simulink model "gm_I2S"  (R2023b)
settings: Solver=VariableStepAuto  StartTime=0.0  StopTime=10000  RelTol=1e-3
undefined symbols (not defined in the file or in its folder): cnt1_LRCLK, cnt2_SCLK, SH_R
libraries: hdlsllib x10
(part 1 of 5)
settings Model: Creator=31651  LastModifiedBy=31651
settings OptimizationCC: BlockReduction=off  ConditionallyExecuteInputs=off  DefaultParameterBehavior=Inlined
settings DebuggingCC: AlgebraicLoopMsg=error  InheritedTsInSrcMsg=none  ParameterPrecisionLossMsg=none
settings HardwareCC: ProdBitPerPointer=32  ProdBitPerSizeT=32  ProdBitPerPtrDiffT=32  ProdLargestAtomicFloat=None  ProdIntDivRoundTo=Undefined  ProdEndianess=Unspecified  ProdWordSize=32  ProdHWDeviceType=ASIC/FPGA->ASIC/FPGA  TargetBitPerPointer=64  TargetBitPerSizeT=64  TargetBitPerPtrDiffT=64  TargetLongLongMode=on  TargetIntDivRoundTo=Zero  TargetEndianess=LittleEndian  TargetWordSize=64  TargetHWDeviceType=Custom Processor->MATLAB Host Computer  ProdEqTarget=off

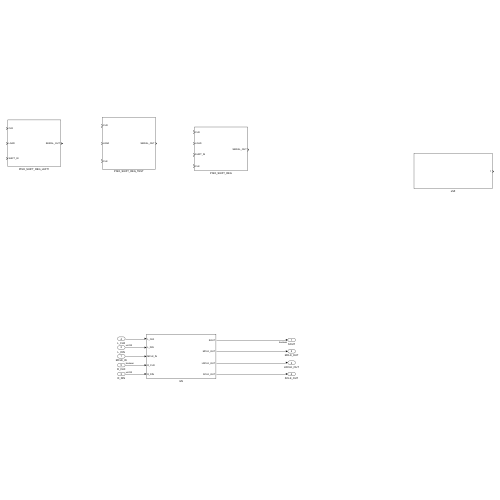
[thumbnail: Simulink's stored preview of the top-level diagram]
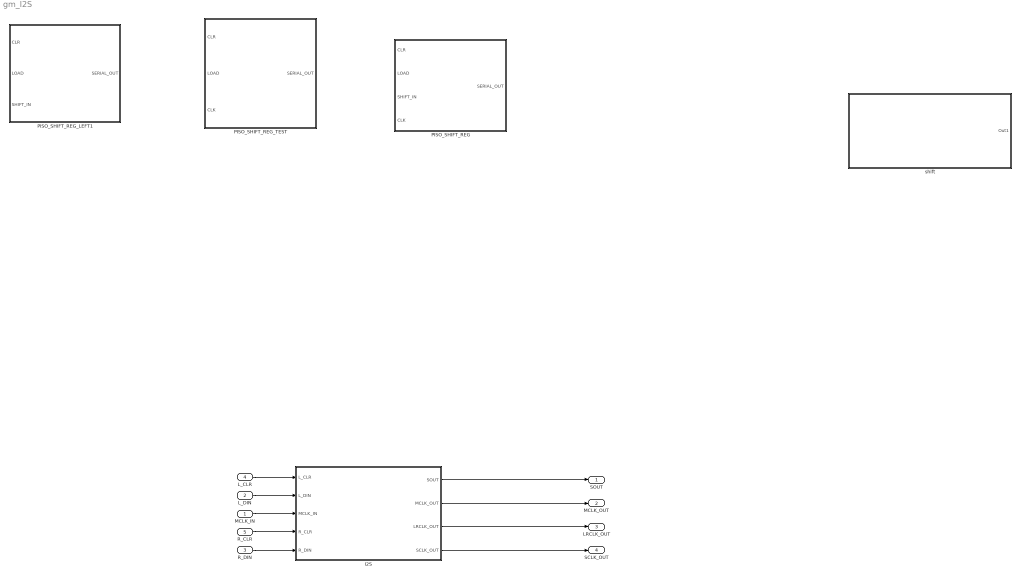
== system gm_I2S ==
  MCLK_IN : Inport
  L_DIN : Inport  Port=2  OutDataTypeStr=uint32
  R_DIN : Inport  Port=3  OutDataTypeStr=uint32
  L_CLR : Inport  Port=4
  R_CLR : Inport  Port=5  OutDataTypeStr=boolean
  I2S : Subsystem
  PISO_SHIFT_REG : Subsystem
  PISO_SHIFT_REG_LEFT1 : Subsystem
  PISO_SHIFT_REG_TEST : Subsystem
  shift : Subsystem
  SOUT : Outport  OutDataTypeStr=boolean  VectorParamsAs1DForOutWhenUnconnected=off
  MCLK_OUT : Outport  Port=2  VectorParamsAs1DForOutWhenUnconnected=off
  LRCLK_OUT : Outport  Port=3  VectorParamsAs1DForOutWhenUnconnected=off
  SCLK_OUT : Outport  Port=4  VectorParamsAs1DForOutWhenUnconnected=off
  wires:
  R_CLR/1 -> I2S/4(R_CLR)
  L_CLR/1 -> I2S/1(L_CLR)
  I2S/4(SCLK_OUT) -> SCLK_OUT/1
  I2S/3(LRCLK_OUT) -> LRCLK_OUT/1
  I2S/2(MCLK_OUT) -> MCLK_OUT/1
  I2S/1(SOUT) -> SOUT/1
  R_DIN/1 -> I2S/5(R_DIN)
  MCLK_IN/1 -> I2S/3(MCLK_IN)
  L_DIN/1 -> I2S/2(L_DIN)

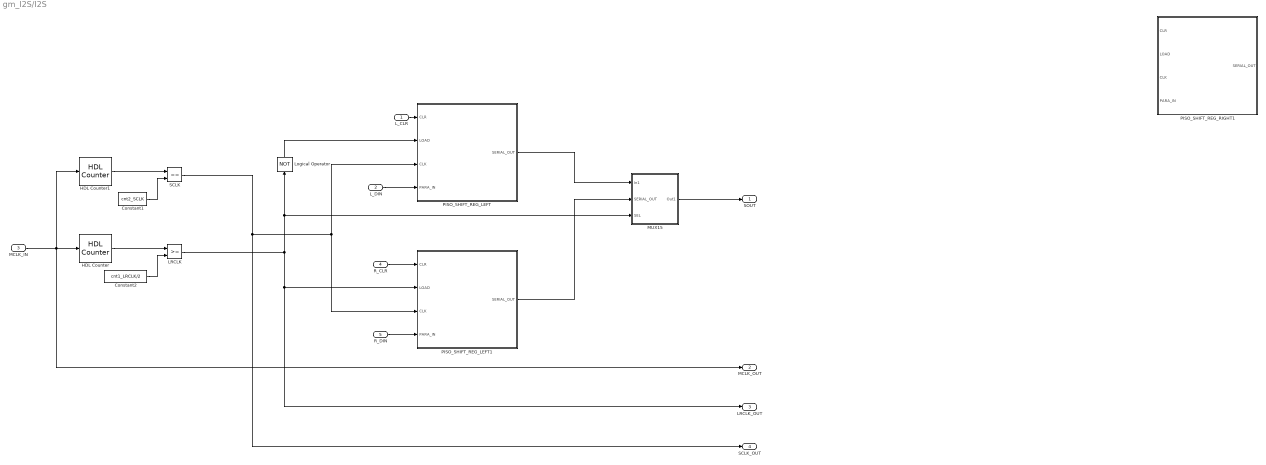
== system gm_I2S/I2S ==
  L_CLR : Inport
  L_DIN : Inport  Port=2
  MCLK_IN : Inport  Port=3
  R_CLR : Inport  Port=4
  R_DIN : Inport  Port=5
  Constant1 : Constant  Value=cnt2_SCLK  OutDataTypeStr=uint16
  Constant2 : Constant  Value=cnt1_LRCLK/2  OutDataTypeStr=uint16
  HDL Counter : hdlsllib/Sources/HDL Counter  CountType=Count limited  CountInit=0  CountStep=1  CountMax=cnt1_LRCLK  CountFromType=Initial value  CountFrom=0  CountResetPort=off  CountLoadPort=off  CountEnbPort=on  CountDirPort=off  CountHitOutputPort=off  CountDataType=Unsigned  CountWordLen=16  CountFracLen=0  CountSampTime=1
  HDL Counter1 : hdlsllib/Sources/HDL Counter  CountType=Count limited  CountInit=0  CountStep=1  CountMax=cnt2_SCLK  CountFromType=Initial value  CountFrom=0  CountResetPort=off  CountLoadPort=off  CountEnbPort=on  CountDirPort=off  CountHitOutputPort=off  CountDataType=Unsigned  CountWordLen=16  CountFracLen=0  CountSampTime=1
  LRCLK : RelationalOperator  OutDataTypeStr=boolean  InputSameDT=off
  Logical Operator : Logic  Operator=NOT  AllPortsSameDT=off  OutDataTypeStr=boolean
  MUX15 : Subsystem
  PISO_SHIFT_REG_LEFT : Subsystem
  PISO_SHIFT_REG_LEFT1 : Subsystem
  PISO_SHIFT_REG_RIGHT1 : Subsystem
  SCLK : RelationalOperator  Operator===  OutDataTypeStr=boolean  InputSameDT=off
  SOUT : Outport  VectorParamsAs1DForOutWhenUnconnected=off
  MCLK_OUT : Outport  Port=2  VectorParamsAs1DForOutWhenUnconnected=off
  LRCLK_OUT : Outport  Port=3  VectorParamsAs1DForOutWhenUnconnected=off
  SCLK_OUT : Outport  Port=4  VectorParamsAs1DForOutWhenUnconnected=off
  wires:
  L_DIN/1 -> PISO_SHIFT_REG_LEFT/4(PARA_IN)
  R_DIN/1 -> PISO_SHIFT_REG_LEFT1/4(PARA_IN)
  L_CLR/1 -> PISO_SHIFT_REG_LEFT/1(CLR)
  Constant2/1 -> LRCLK/2
  HDL Counter1/1 -> SCLK/1
  R_CLR/1 -> PISO_SHIFT_REG_LEFT1/1(CLR)
  MUX15/1(Out1) -> SOUT/1
  Constant1/1 -> SCLK/2
  PISO_SHIFT_REG_LEFT1/1(SERIAL_OUT) -> MUX15/2(SERIAL_OUT)
  MCLK_IN/1 -> HDL Counter/1, HDL Counter1/1, MCLK_OUT/1
  HDL Counter/1 -> LRCLK/1
  PISO_SHIFT_REG_LEFT/1(SERIAL_OUT) -> MUX15/1(In1)
  LRCLK/1 -> MUX15/3(SEL), Logical Operator/1, LRCLK_OUT/1, PISO_SHIFT_REG_LEFT1/2(LOAD)
  Logical Operator/1 -> PISO_SHIFT_REG_LEFT/2(LOAD)
  SCLK/1 -> PISO_SHIFT_REG_LEFT/3(CLK), PISO_SHIFT_REG_LEFT1/3(CLK), SCLK_OUT/1

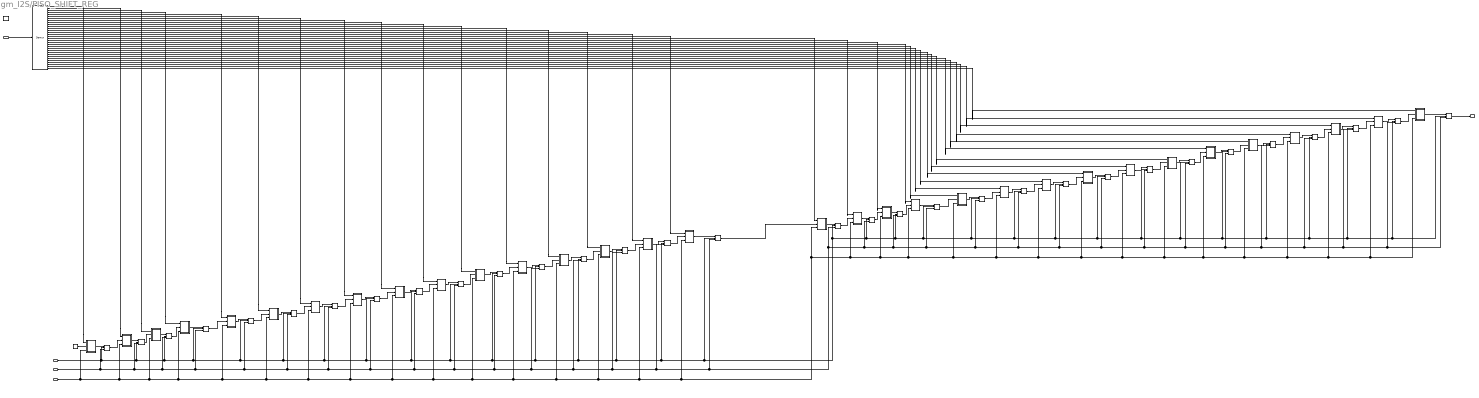
== system gm_I2S/PISO_SHIFT_REG ==
  note: LOAD=0写入数据
      | LOAD=1 移位
      | 边沿清零
  CLR : Inport
  LOAD : Inport  Port=2
  SHIFT_IN : Inport  Port=3
  CLK : Inport  Port=4  OutDataTypeStr=boolean
  Constant : Constant  Value=SH_R
  Constant5 : Constant  Value=0  OutDataTypeStr=boolean  SampleTime=1
  Delay{,1..15,17..24,26..33} (32 alike) : Delay  DelayLength=1  ExternalReset=Either  ShowEnablePort=on
      settings: InputPortMap=u0,e6,r5
  Demux : Demux  Outputs=32
      settings: DisplayOption=none
  MUX : Subsystem
  MUX1 : Subsystem
  MUX10 : Subsystem
  MUX11 : Subsystem
  MUX12 : Subsystem
  MUX13 : Subsystem
  MUX14 : Subsystem
  MUX15 : Subsystem
  MUX16 : Subsystem
  MUX17 : Subsystem
  MUX18 : Subsystem
  MUX19 : Subsystem
  MUX2 : Subsystem
  MUX20 : Subsystem
  MUX21 : Subsystem
  MUX22 : Subsystem
  MUX23 : Subsystem
  MUX24 : Subsystem
  MUX25 : Subsystem
  MUX26 : Subsystem
  MUX27 : Subsystem
  MUX28 : Subsystem
  MUX29 : Subsystem
  MUX3 : Subsystem
  MUX30 : Subsystem
  MUX31 : Subsystem
  MUX4 : Subsystem
  MUX5 : Subsystem
  MUX6 : Subsystem
  MUX7 : Subsystem
  MUX8 : Subsystem
  MUX9 : Subsystem
  SERIAL_OUT : Outport  VectorParamsAs1DForOutWhenUnconnected=off
  wires:
  SHIFT_IN/1 -> Demux/1
  Demux/19 -> MUX24/1(In1)
  MUX22/1(Out1) -> Delay23/1
  MUX19/1(Out1) -> Delay20/1
  Delay30/1 -> MUX29/2(In2)
  MUX24/1(Out1) -> Delay26/1
  MUX21/1(Out1) -> Delay22/1
  Demux/32 -> MUX23/1(In1)
  Delay23/1 -> MUX23/2(In2)
  Delay22/1 -> MUX22/2(In2)
  Delay33/1 -> MUX18/2(In2)
  Delay15/1 -> MUX16/2(In2)
  MUX23/1(Out1) -> Delay24/1
  MUX28/1(Out1) -> Delay30/1
  Delay19/1 -> MUX19/2(In2)
  MUX18/1(Out1) -> Delay19/1
  Delay20/1 -> MUX20/2(In2)
  MUX26/1(Out1) -> Delay28/1
  Delay27/1 -> MUX26/2(In2)
  Demux/25 -> MUX30/1(In1)
  Demux/31 -> MUX22/1(In1)
  Demux/21 -> MUX26/1(In1)
  Delay18/1 -> MUX24/2(In2)
  Demux/17 -> MUX16/1(In1)
  Demux/18 -> MUX17/1(In1)
  Demux/29 -> MUX20/1(In1)
  CLR/1 -> Delay1/3, Delay2/3, Delay3/3, Delay4/3, Delay5/3, Delay6/3, Delay7/3, Delay8/3, Delay9/3, Delay10/3, Delay11/3, Delay12/3, Delay13/3, Delay14/3, Delay15/3, Delay17/3, Delay18/3, Delay26/3, Delay27/3, Delay28/3, Delay29/3, Delay30/3, Delay31/3, Delay32/3, Delay33/3, Delay19/3, Delay20/3, Delay21/3, Delay22/3, Delay23/3, Delay24/3, Delay/3
  Demux/20 -> MUX25/1(In1)
  Delay24/1 -> SERIAL_OUT/1
  Demux/26 -> MUX31/1(In1)
  MUX20/1(Out1) -> Delay21/1
  Delay21/1 -> MUX21/2(In2)
  MUX27/1(Out1) -> Delay29/1
  Demux/22 -> MUX27/1(In1)
  Delay28/1 -> MUX27/2(In2)
  Delay29/1 -> MUX28/2(In2)
  Demux/23 -> MUX28/1(In1)
  MUX16/1(Out1) -> Delay17/1
  Delay17/1 -> MUX17/2(In2)
  MUX17/1(Out1) -> Delay18/1
  Delay32/1 -> MUX31/2(In2)
  Delay31/1 -> MUX30/2(In2)
  MUX30/1(Out1) -> Delay32/1
  MUX29/1(Out1) -> Delay31/1
  MUX31/1(Out1) -> Delay33/1
  LOAD/1 -> MUX2/3(SEL), MUX3/3(SEL), MUX24/3(SEL), MUX25/3(SEL), MUX23/3(SEL), MUX22/3(SEL), MUX21/3(SEL), MUX20/3(SEL), MUX19/3(SEL), MUX18/3(SEL), MUX31/3(SEL), MUX30/3(SEL), MUX29/3(SEL), MUX28/3(SEL), MUX27/3(SEL), MUX26/3(SEL), MUX17/3(SEL), MUX16/3(SEL), MUX15/3(SEL), MUX14/3(SEL), MUX13/3(SEL), MUX12/3(SEL), MUX11/3(SEL), MUX10/3(SEL), MUX9/3(SEL), MUX8/3(SEL), MUX7/3(SEL), MUX6/3(SEL), MUX5/3(SEL), MUX4/3(SEL), MUX1/3(SEL), MUX/3(SEL)
  MUX25/1(Out1) -> Delay27/1
  Delay26/1 -> MUX25/2(In2)
  Demux/27 -> MUX18/1(In1)
  Demux/28 -> MUX19/1(In1)
  Demux/24 -> MUX29/1(In1)
  CLK/1 -> Delay3/2, Delay4/2, Delay5/2, Delay6/2, Delay7/2, Delay9/2, Delay27/2, Delay28/2, Delay29/2, Delay30/2, Delay31/2, Delay33/2, Delay24/2, Delay23/2, Delay22/2, Delay21/2, Delay20/2, Delay19/2, Delay32/2, Delay26/2, Delay18/2, Delay17/2, Delay15/2, Delay14/2, Delay13/2, Delay12/2, Delay11/2, Delay10/2, Delay8/2, Delay2/2, Delay1/2, Delay/2
  Demux/30 -> MUX21/1(In1)
  Demux/16 -> MUX15/1(In1)
  Demux/15 -> MUX14/1(In1)
  Demux/14 -> MUX13/1(In1)
  Demux/13 -> MUX12/1(In1)
  Demux/12 -> MUX11/1(In1)
  Demux/11 -> MUX10/1(In1)
  Demux/10 -> MUX9/1(In1)
  Demux/9 -> MUX8/1(In1)
  Demux/8 -> MUX7/1(In1)
  Demux/7 -> MUX6/1(In1)
  Demux/6 -> MUX5/1(In1)
  Demux/5 -> MUX4/1(In1)
  Delay12/1 -> MUX13/2(In2)
  Delay9/1 -> MUX10/2(In2)
  Delay6/1 -> MUX7/2(In2)
  MUX13/1(Out1) -> Delay13/1
  MUX15/1(Out1) -> Delay15/1
  MUX14/1(Out1) -> Delay14/1
  Delay13/1 -> MUX14/2(In2)
  Delay14/1 -> MUX15/2(In2)
  MUX10/1(Out1) -> Delay10/1
  MUX12/1(Out1) -> Delay12/1
  MUX11/1(Out1) -> Delay11/1
  Delay10/1 -> MUX11/2(In2)
  Delay11/1 -> MUX12/2(In2)
  MUX7/1(Out1) -> Delay7/1
  MUX9/1(Out1) -> Delay9/1
  MUX8/1(Out1) -> Delay8/1
  Delay7/1 -> MUX8/2(In2)
  Delay8/1 -> MUX9/2(In2)
  Delay5/1 -> MUX6/2(In2)
  Delay4/1 -> MUX5/2(In2)
  Delay3/1 -> MUX4/2(In2)
  MUX6/1(Out1) -> Delay6/1
  MUX5/1(Out1) -> Delay5/1
  MUX4/1(Out1) -> Delay4/1
  Demux/1 -> MUX/1(In1)
  Constant5/1 -> MUX/2(In2)
  MUX3/1(Out1) -> Delay3/1
  Delay2/1 -> MUX3/2(In2)
  Demux/4 -> MUX3/1(In1)
  Delay1/1 -> MUX2/2(In2)
  Demux/3 -> MUX2/1(In1)
  MUX2/1(Out1) -> Delay2/1
  Delay/1 -> MUX1/2(In2)
  MUX1/1(Out1) -> Delay1/1
  Demux/2 -> MUX1/1(In1)
  MUX/1(Out1) -> Delay/1

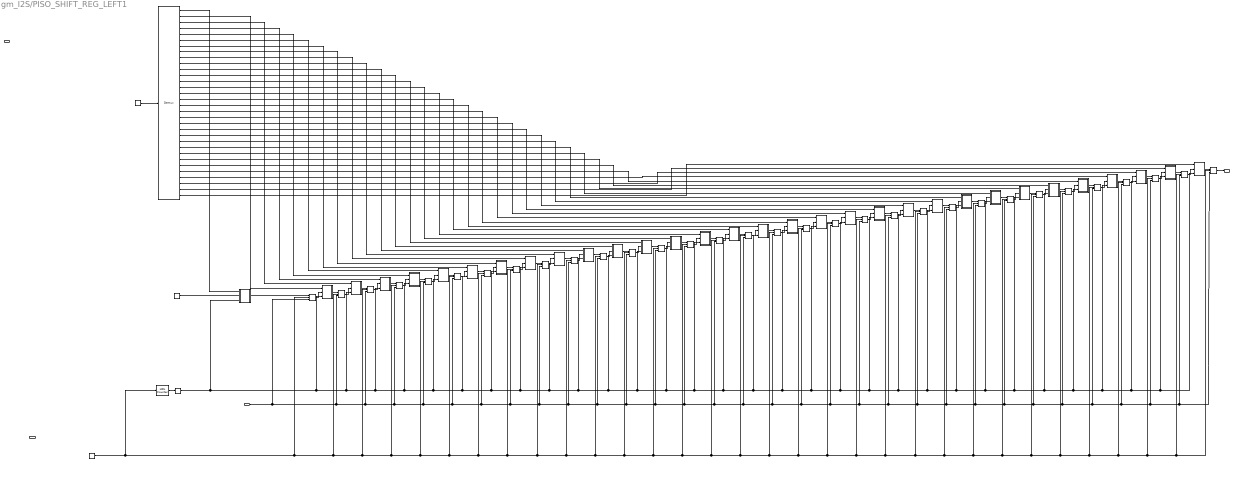
== system gm_I2S/PISO_SHIFT_REG_LEFT1 ==
  note: LOAD=0写入数据
      | LOAD=1 移位
      | 边沿清零
  CLR : Inport
  LOAD : Inport  Port=2
  SHIFT_IN : Inport  Port=3
  Compare To Constant : hdlsllib/Logic and Bit Operations/Compare To Constant  relop=>=  const=5  OutDataTypeStr=boolean
  Constant : Constant  Value=SH_R
  Constant1 : Constant  OutDataTypeStr=boolean  SampleTime=1
  Constant5 : Constant  Value=0  OutDataTypeStr=boolean  SampleTime=1
  Delay{,1..15,17..24,26..33} (32 alike) : Delay  DelayLength=1  ExternalReset=Either  ShowEnablePort=on
      settings: InputPortMap=u0,e6,r5
  Demux : Demux  Outputs=32
      settings: DisplayOption=none
  HDL Counter : hdlsllib/Sources/HDL Counter  CountType=Count limited  CountInit=0  CountStep=1  CountMax=10000  CountFromType=Initial value  CountFrom=0  CountResetPort=off  CountLoadPort=off  CountEnbPort=on  CountDirPort=off  CountHitOutputPort=off  CountDataType=Unsigned  CountWordLen=16  CountFracLen=0  CountSampTime=1
  MUX : Subsystem
  MUX1 : Subsystem
  MUX10 : Subsystem
  MUX11 : Subsystem
  MUX12 : Subsystem
  MUX13 : Subsystem
  MUX14 : Subsystem
  MUX15 : Subsystem
  MUX16 : Subsystem
  MUX17 : Subsystem
  MUX18 : Subsystem
  MUX19 : Subsystem
  MUX2 : Subsystem
  MUX20 : Subsystem
  MUX21 : Subsystem
  MUX22 : Subsystem
  MUX23 : Subsystem
  MUX24 : Subsystem
  MUX25 : Subsystem
  MUX26 : Subsystem
  MUX27 : Subsystem
  MUX28 : Subsystem
  MUX29 : Subsystem
  MUX3 : Subsystem
  MUX30 : Subsystem
  MUX31 : Subsystem
  MUX4 : Subsystem
  MUX5 : Subsystem
  MUX6 : Subsystem
  MUX7 : Subsystem
  MUX8 : Subsystem
  MUX9 : Subsystem
  SERIAL_OUT : Outport  VectorParamsAs1DForOutWhenUnconnected=off
  wires:
  Demux/2 -> MUX1/1(In1)
  Demux/3 -> MUX2/1(In1)
  Demux/4 -> MUX3/1(In1)
  Demux/6 -> MUX5/1(In1)
  Demux/7 -> MUX6/1(In1)
  Demux/9 -> MUX8/1(In1)
  Demux/11 -> MUX10/1(In1)
  Demux/12 -> MUX11/1(In1)
  Demux/13 -> MUX12/1(In1)
  Demux/15 -> MUX14/1(In1)
  Demux/14 -> MUX13/1(In1)
  Demux/24 -> MUX29/1(In1)
  Demux/10 -> MUX9/1(In1)
  Demux/28 -> MUX19/1(In1)
  Demux/27 -> MUX18/1(In1)
  Demux/22 -> MUX27/1(In1)
  Demux/30 -> MUX21/1(In1)
  Demux/26 -> MUX31/1(In1)
  Demux/5 -> MUX4/1(In1)
  Demux/20 -> MUX25/1(In1)
  Demux/21 -> MUX26/1(In1)
  Demux/31 -> MUX22/1(In1)
  Demux/25 -> MUX30/1(In1)
  Demux/17 -> MUX16/1(In1)
  Demux/32 -> MUX23/1(In1)
  Demux/18 -> MUX17/1(In1)
  Demux/19 -> MUX24/1(In1)
  Demux/23 -> MUX28/1(In1)
  Demux/16 -> MUX15/1(In1)
  Demux/29 -> MUX20/1(In1)
  Demux/8 -> MUX7/1(In1)
  Constant1/1 -> HDL Counter/1, Delay/2, Delay1/2, Delay2/2, Delay3/2, Delay4/2, Delay5/2, Delay6/2, Delay7/2, Delay8/2, Delay9/2, Delay10/2, Delay11/2, Delay12/2, Delay13/2, Delay14/2, Delay15/2, Delay17/2, Delay18/2, Delay26/2, Delay27/2, Delay28/2, Delay29/2, Delay30/2, Delay31/2, Delay32/2, Delay33/2, Delay19/2, Delay20/2, Delay21/2, Delay22/2, Delay23/2, Delay24/2
  CLR/1 -> Delay/3, Delay1/3, Delay2/3, Delay3/3, Delay4/3, Delay5/3, Delay6/3, Delay7/3, Delay8/3, Delay9/3, Delay10/3, Delay11/3, Delay12/3, Delay13/3, Delay14/3, Delay15/3, Delay17/3, Delay18/3, Delay26/3, Delay27/3, Delay28/3, Delay29/3, Delay30/3, Delay31/3, Delay32/3, Delay33/3, Delay19/3, Delay20/3, Delay21/3, Delay22/3, Delay23/3, Delay24/3
  MUX1/1(Out1) -> Delay1/1
  Delay/1 -> MUX1/2(In2)
  MUX2/1(Out1) -> Delay2/1
  Delay1/1 -> MUX2/2(In2)
  Demux/1 -> MUX/1(In1)
  MUX6/1(Out1) -> Delay6/1
  Compare To Constant/1 -> MUX/3(SEL), MUX1/3(SEL), MUX2/3(SEL), MUX3/3(SEL), MUX4/3(SEL), MUX5/3(SEL), MUX6/3(SEL), MUX7/3(SEL), MUX8/3(SEL), MUX9/3(SEL), MUX10/3(SEL), MUX11/3(SEL), MUX12/3(SEL), MUX13/3(SEL), MUX14/3(SEL), MUX15/3(SEL), MUX16/3(SEL), MUX17/3(SEL), MUX24/3(SEL), MUX25/3(SEL), MUX26/3(SEL), MUX27/3(SEL), MUX28/3(SEL), MUX29/3(SEL), MUX30/3(SEL), MUX31/3(SEL), MUX18/3(SEL), MUX19/3(SEL), MUX20/3(SEL), MUX21/3(SEL), MUX23/3(SEL), MUX22/3(SEL)
  Delay7/1 -> MUX8/2(In2)
  Delay11/1 -> MUX12/2(In2)
  MUX11/1(Out1) -> Delay11/1
  Delay2/1 -> MUX3/2(In2)
  MUX10/1(Out1) -> Delay10/1
  Delay13/1 -> MUX14/2(In2)
  MUX5/1(Out1) -> Delay5/1
  Constant5/1 -> MUX/2(In2)
  MUX8/1(Out1) -> Delay8/1
  MUX14/1(Out1) -> Delay14/1
  MUX15/1(Out1) -> Delay15/1
  Delay6/1 -> MUX7/2(In2)
  Delay9/1 -> MUX10/2(In2)
  MUX12/1(Out1) -> Delay12/1
  MUX7/1(Out1) -> Delay7/1
  MUX31/1(Out1) -> Delay33/1
  MUX3/1(Out1) -> Delay3/1
  MUX16/1(Out1) -> Delay17/1
  Delay28/1 -> MUX27/2(In2)
  Delay12/1 -> MUX13/2(In2)
  Delay21/1 -> MUX21/2(In2)
  Delay18/1 -> MUX24/2(In2)
  Delay31/1 -> MUX30/2(In2)
  MUX17/1(Out1) -> Delay18/1
  Delay20/1 -> MUX20/2(In2)
  Delay19/1 -> MUX19/2(In2)
  MUX28/1(Out1) -> Delay30/1
  MUX30/1(Out1) -> Delay32/1
  MUX13/1(Out1) -> Delay13/1
  MUX23/1(Out1) -> Delay24/1
  Delay3/1 -> MUX4/2(In2)
  Delay5/1 -> MUX6/2(In2)
  MUX26/1(Out1) -> Delay28/1
  Delay8/1 -> MUX9/2(In2)
  Delay33/1 -> MUX18/2(In2)
  MUX25/1(Out1) -> Delay27/1
  Delay24/1 -> SERIAL_OUT/1
  Delay17/1 -> MUX17/2(In2)
  Delay10/1 -> MUX11/2(In2)
  MUX27/1(Out1) -> Delay29/1
  Delay15/1 -> MUX16/2(In2)
  Delay22/1 -> MUX22/2(In2)
  Delay32/1 -> MUX31/2(In2)
  Delay4/1 -> MUX5/2(In2)
  Delay23/1 -> MUX23/2(In2)
  MUX20/1(Out1) -> Delay21/1
  Delay29/1 -> MUX28/2(In2)
  Delay27/1 -> MUX26/2(In2)
  Delay30/1 -> MUX29/2(In2)
  Delay26/1 -> MUX25/2(In2)
  MUX24/1(Out1) -> Delay26/1
  MUX4/1(Out1) -> Delay4/1
  MUX21/1(Out1) -> Delay22/1
  MUX29/1(Out1) -> Delay31/1
  MUX18/1(Out1) -> Delay19/1
  MUX9/1(Out1) -> Delay9/1
  MUX/1(Out1) -> Delay/1
  MUX22/1(Out1) -> Delay23/1
  Delay14/1 -> MUX15/2(In2)
  Constant/1 -> Demux/1
  MUX19/1(Out1) -> Delay20/1
  HDL Counter/1 -> Compare To Constant/1

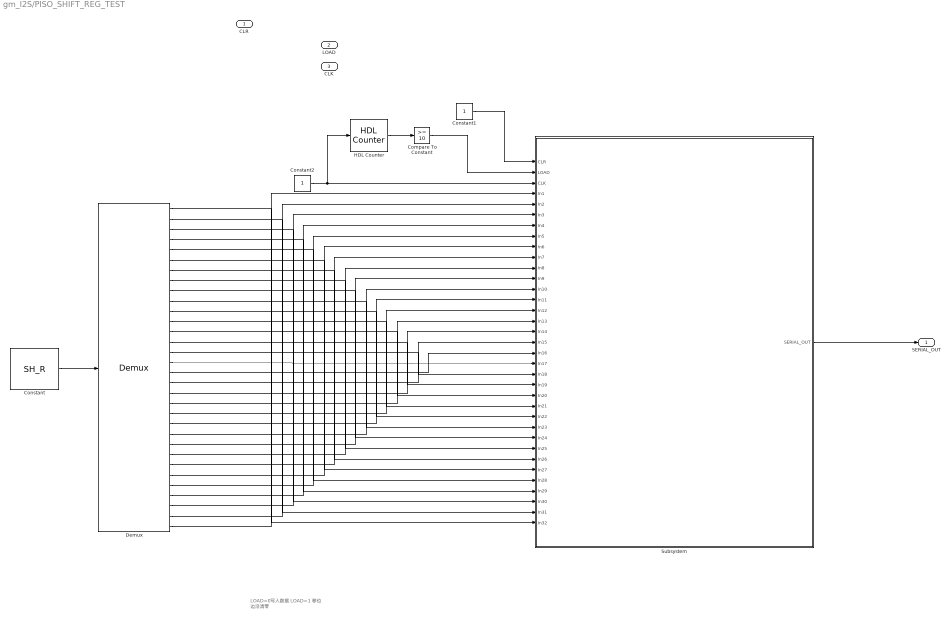
== system gm_I2S/PISO_SHIFT_REG_TEST ==
  note: LOAD=0写入数据
      | LOAD=1 移位
      | 边沿清零
  CLR : Inport
  LOAD : Inport  Port=2
  CLK : Inport  Port=3
  Compare To Constant : hdlsllib/Logic and Bit Operations/Compare To Constant  relop=>=  const=10  OutDataTypeStr=boolean
  Constant : Constant  Value=SH_R  SampleTime=1
  Constant1 : Constant  OutDataTypeStr=boolean
  Constant2 : Constant  OutDataTypeStr=boolean  SampleTime=1
  Demux : Demux  Outputs=32
      settings: DisplayOption=none
  HDL Counter : hdlsllib/Sources/HDL Counter  CountType=Count limited  CountInit=0  CountStep=1  CountMax=10000  CountFromType=Initial value  CountFrom=0  CountResetPort=off  CountLoadPort=off  CountEnbPort=on  CountDirPort=off  CountHitOutputPort=off  CountDataType=Unsigned  CountWordLen=16  CountFracLen=0  CountSampTime=1
  Subsystem : Subsystem
  SERIAL_OUT : Outport  VectorParamsAs1DForOutWhenUnconnected=off
  wires:
  Compare To Constant/1 -> Subsystem/2(LOAD)
  HDL Counter/1 -> Compare To Constant/1
  Constant2/1 -> Subsystem/3(CLK), HDL Counter/1
  Constant1/1 -> Subsystem/1(CLR)
  Constant/1 -> Demux/1
  Demux/29 -> Subsystem/7(In4)
  Demux/28 -> Subsystem/8(In5)
  Demux/27 -> Subsystem/9(In6)
  Demux/26 -> Subsystem/10(In7)
  Demux/25 -> Subsystem/11(In8)
  Demux/24 -> Subsystem/12(In9)
  Demux/23 -> Subsystem/13(In10)
  Demux/22 -> Subsystem/14(In11)
  Demux/21 -> Subsystem/15(In12)
  Demux/20 -> Subsystem/16(In13)
  Demux/19 -> Subsystem/17(In14)
  Demux/18 -> Subsystem/18(In15)
  Demux/30 -> Subsystem/6(In3)
  Demux/31 -> Subsystem/5(In2)
  Demux/32 -> Subsystem/4(In1)
  Demux/17 -> Subsystem/19(In16)
  Demux/16 -> Subsystem/20(In17)
  Demux/15 -> Subsystem/21(In18)
  Demux/14 -> Subsystem/22(In19)
  Demux/13 -> Subsystem/23(In20)
  Demux/12 -> Subsystem/24(In21)
  Demux/11 -> Subsystem/25(In22)
  Demux/10 -> Subsystem/26(In23)
  Demux/9 -> Subsystem/27(In24)
  Demux/8 -> Subsystem/28(In25)
  Demux/7 -> Subsystem/29(In26)
  Demux/6 -> Subsystem/30(In27)
  Demux/5 -> Subsystem/31(In28)
  Demux/4 -> Subsystem/32(In29)
  Demux/3 -> Subsystem/33(In30)
  Demux/2 -> Subsystem/34(In31)
  Demux/1 -> Subsystem/35(In32)
  Subsystem/1(SERIAL_OUT) -> SERIAL_OUT/1

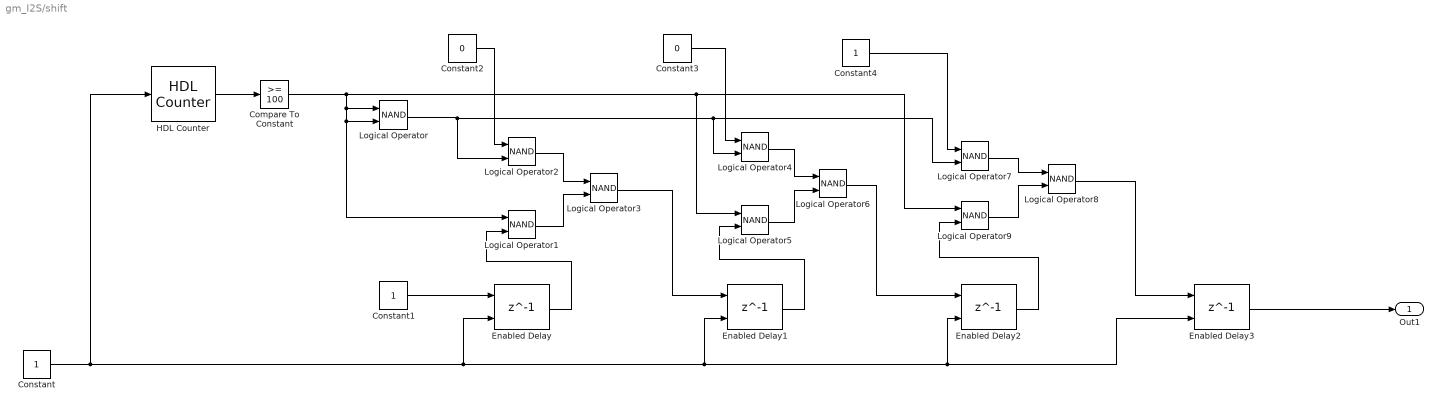
== system gm_I2S/shift ==
  Compare To Constant : hdlsllib/Logic and Bit Operations/Compare To Constant  relop=>=  const=100  OutDataTypeStr=boolean
  Constant : Constant  OutDataTypeStr=boolean  SampleTime=1
  Constant1 : Constant  OutDataTypeStr=boolean  SampleTime=1
  Constant2 : Constant  Value=0  OutDataTypeStr=boolean  SampleTime=1
  Constant3 : Constant  Value=0  OutDataTypeStr=boolean  SampleTime=1
  Constant4 : Constant  OutDataTypeStr=boolean  SampleTime=1
  Enabled Delay{,1..3} (4 alike) : Delay  DelayLength=1  ShowEnablePort=on
      settings: InputPortMap=u0,e6
  HDL Counter : hdlsllib/Sources/HDL Counter  CountType=Count limited  CountInit=0  CountStep=1  CountMax=1000  CountFromType=Initial value  CountFrom=0  CountResetPort=off  CountLoadPort=off  CountEnbPort=on  CountDirPort=off  CountHitOutputPort=off  CountDataType=Unsigned  CountWordLen=16  CountFracLen=0  CountSampTime=1
  Logical Operator{,1..9} (10 alike) : Logic  Operator=NAND  AllPortsSameDT=off  OutDataTypeStr=boolean
  Out1 : Outport  VectorParamsAs1DForOutWhenUnconnected=off
  wires:
  HDL Counter/1 -> Compare To Constant/1
  Constant1/1 -> Enabled Delay/1
  Enabled Delay3/1 -> Out1/1
  Constant4/1 -> Logical Operator7/1
  Constant3/1 -> Logical Operator4/1
  Constant2/1 -> Logical Operator2/1
  Constant/1 -> Enabled Delay2/2, Enabled Delay3/2, Enabled Delay1/2, Enabled Delay/2, HDL Counter/1
  Logical Operator8/1 -> Enabled Delay3/1
  Logical Operator6/1 -> Enabled Delay2/1
  Enabled Delay2/1 -> Logical Operator9/2
  Logical Operator9/1 -> Logical Operator8/2
  Logical Operator7/1 -> Logical Operator8/1
  Enabled Delay1/1 -> Logical Operator5/2
  Logical Operator3/1 -> Enabled Delay1/1
  Logical Operator4/1 -> Logical Operator6/1
  Logical Operator5/1 -> Logical Operator6/2
  Compare To Constant/1 -> Logical Operator/1, Logical Operator/2, Logical Operator1/1, Logical Operator5/1, Logical Operator9/1
  Enabled Delay/1 -> Logical Operator1/2
  Logical Operator/1 -> Logical Operator4/2, Logical Operator7/2, Logical Operator2/2
  Logical Operator2/1 -> Logical Operator3/1
  Logical Operator1/1 -> Logical Operator3/2

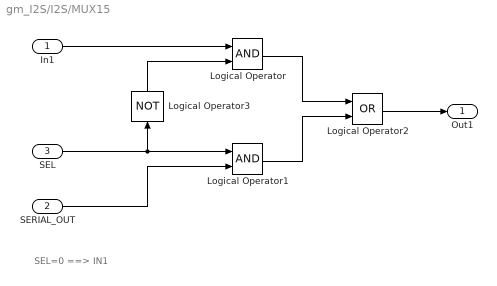
== system gm_I2S/I2S/MUX15 ==
  note: SEL=0 ==> IN1
  In1 : Inport
  SERIAL_OUT : Inport  Port=2
  SEL : Inport  Port=3  OutDataTypeStr=boolean
  Logical Operator : Logic  AllPortsSameDT=off  OutDataTypeStr=boolean
  Logical Operator1 : Logic  AllPortsSameDT=off  OutDataTypeStr=boolean
  Logical Operator2 : Logic  Operator=OR  AllPortsSameDT=off  OutDataTypeStr=boolean
  Logical Operator3 : Logic  Operator=NOT  AllPortsSameDT=off  OutDataTypeStr=boolean
  Out1 : Outport  VectorParamsAs1DForOutWhenUnconnected=off
  wires:
  SERIAL_OUT/1 -> Logical Operator1/2
  Logical Operator2/1 -> Out1/1
  Logical Operator/1 -> Logical Operator2/1
  Logical Operator1/1 -> Logical Operator2/2
  Logical Operator3/1 -> Logical Operator/2
  SEL/1 -> Logical Operator1/1, Logical Operator3/1
  In1/1 -> Logical Operator/1

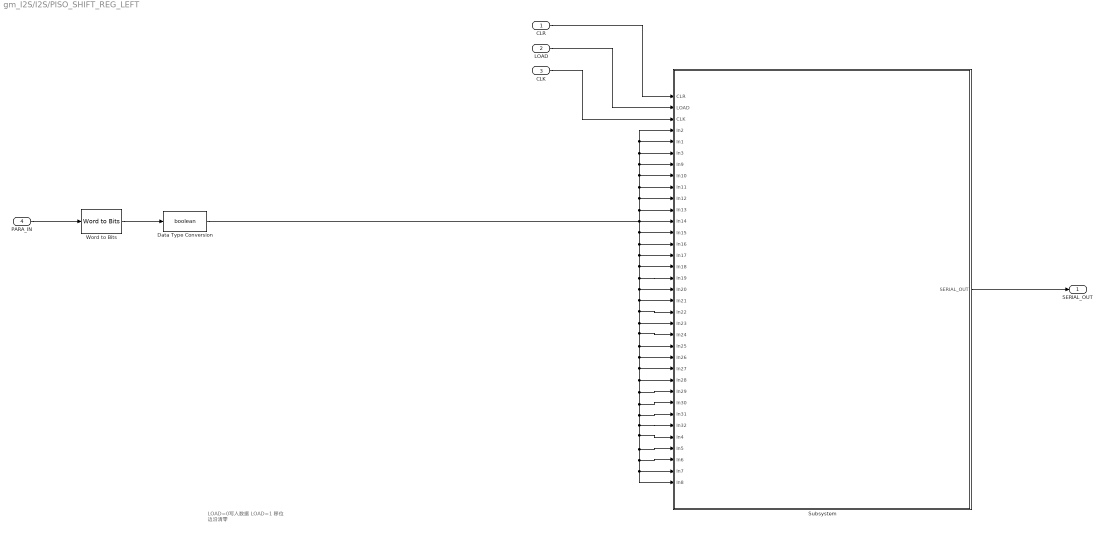
== system gm_I2S/I2S/PISO_SHIFT_REG_LEFT ==
  note: LOAD=0写入数据
      | LOAD=1 移位
      | 边沿清零
  CLR : Inport
  LOAD : Inport  Port=2
  CLK : Inport  Port=3
  PARA_IN : Inport  Port=4  OutDataTypeStr=uint32
  Data Type Conversion : DataTypeConversion  OutDataTypeStr=boolean  SaturateOnIntegerOverflow=off  RndMeth=Floor
  Subsystem : Subsystem
  Word to Bits : hdlsllib/Logic and Bit Operations/Word to Bits  maxWordLength=32
  SERIAL_OUT : Outport  OutDataTypeStr=boolean  VectorParamsAs1DForOutWhenUnconnected=off
  wires:
  Data Type Conversion/1 -> Subsystem/12(In14), Subsystem/15(In17), Subsystem/18(In20), Subsystem/35(In8), Subsystem/34(In7), Subsystem/33(In6), Subsystem/32(In5), Subsystem/31(In4), Subsystem/30(In32), Subsystem/29(In31), Subsystem/28(In30), Subsystem/27(In29), Subsystem/26(In28), Subsystem/25(In27), Subsystem/24(In26), Subsystem/23(In25), Subsystem/22(In24), Subsystem/21(In23), Subsystem/20(In22), Subsystem/19(In21), Subsystem/17(In19), Subsystem/16(In18), Subsystem/14(In16), Subsystem/13(In15), Subsystem/11(In13), Subsystem/9(In11), Subsystem/4(In2), Subsystem/5(In1), Subsystem/6(In3), Subsystem/7(In9), Subsystem/8(In10), Subsystem/10(In12)
  Word to Bits/1 -> Data Type Conversion/1
  PARA_IN/1 -> Word to Bits/1
  CLR/1 -> Subsystem/1(CLR)
  LOAD/1 -> Subsystem/2(LOAD)
  CLK/1 -> Subsystem/3(CLK)
  Subsystem/1(SERIAL_OUT) -> SERIAL_OUT/1

== system gm_I2S/I2S/PISO_SHIFT_REG_LEFT1 ==
  note: LOAD=0写入数据
      | LOAD=1 移位
      | 边沿清零
  CLR : Inport
  LOAD : Inport  Port=2
  CLK : Inport  Port=3
  PARA_IN : Inport  Port=4  OutDataTypeStr=uint32
  Data Type Conversion : DataTypeConversion  OutDataTypeStr=boolean  SaturateOnIntegerOverflow=off  RndMeth=Floor
  Subsystem : Subsystem
  Word to Bits : hdlsllib/Logic and Bit Operations/Word to Bits  maxWordLength=32
  SERIAL_OUT : Outport  OutDataTypeStr=boolean  VectorParamsAs1DForOutWhenUnconnected=off
  wires:
  Data Type Conversion/1 -> Subsystem/12(In14), Subsystem/18(In20), Subsystem/35(In8), Subsystem/34(In7), Subsystem/33(In6), Subsystem/32(In5), Subsystem/31(In4), Subsystem/30(In32), Subsystem/29(In31), Subsystem/28(In30), Subsystem/27(In29), Subsystem/26(In28), Subsystem/25(In27), Subsystem/24(In26), Subsystem/23(In25), Subsystem/22(In24), Subsystem/21(In23), Subsystem/20(In22), Subsystem/19(In21), Subsystem/17(In19), Subsystem/16(In18), Subsystem/15(In17), Subsystem/14(In16), Subsystem/13(In15), Subsystem/11(In13), Subsystem/9(In11), Subsystem/4(In2), Subsystem/5(In1), Subsystem/6(In3), Subsystem/7(In9), Subsystem/8(In10), Subsystem/10(In12)
  Word to Bits/1 -> Data Type Conversion/1
  PARA_IN/1 -> Word to Bits/1
  CLR/1 -> Subsystem/1(CLR)
  LOAD/1 -> Subsystem/2(LOAD)
  CLK/1 -> Subsystem/3(CLK)
  Subsystem/1(SERIAL_OUT) -> SERIAL_OUT/1

== system gm_I2S/I2S/PISO_SHIFT_REG_RIGHT1 ==
  note: LOAD=0写入数据
      | LOAD=1 移位
      | 边沿清零
  CLR : Inport
  LOAD : Inport  Port=2
  CLK : Inport  Port=3
  PARA_IN : Inport  Port=4  OutDataTypeStr=uint32
  Demux : Demux  Outputs=32
      settings: DisplayOption=none
  Subsystem : Subsystem
  SERIAL_OUT : Outport  VectorParamsAs1DForOutWhenUnconnected=off
  wires:
  ? -> Demux/1
  PARA_IN/1 -> ?
  CLR/1 -> Subsystem/1(CLR)
  LOAD/1 -> Subsystem/2(LOAD)
  CLK/1 -> Subsystem/3(CLK)
  Demux/29 -> Subsystem/7(In9)
  Demux/28 -> Subsystem/8(In10)
  Demux/27 -> Subsystem/9(In11)
  Demux/26 -> Subsystem/10(In12)
  Demux/25 -> Subsystem/11(In13)
  Demux/24 -> Subsystem/12(In14)
  Demux/23 -> Subsystem/13(In15)
  Demux/22 -> Subsystem/14(In16)
  Demux/21 -> Subsystem/15(In17)
  Demux/20 -> Subsystem/16(In18)
  Demux/19 -> Subsystem/17(In19)
  Demux/18 -> Subsystem/18(In20)
  Demux/30 -> Subsystem/6(In3)
  Demux/31 -> Subsystem/5(In2)
  Demux/32 -> Subsystem/4(In1)
  Demux/17 -> Subsystem/19(In21)
  Demux/16 -> Subsystem/20(In22)
  Demux/15 -> Subsystem/21(In23)
  Demux/14 -> Subsystem/22(In24)
  Demux/13 -> Subsystem/23(In25)
  Demux/12 -> Subsystem/24(In26)
  Demux/11 -> Subsystem/25(In27)
  Demux/10 -> Subsystem/26(In28)
  Demux/9 -> Subsystem/27(In29)
  Demux/8 -> Subsystem/28(In30)
  Demux/7 -> Subsystem/29(In31)
  Demux/6 -> Subsystem/30(In32)
  Demux/5 -> Subsystem/31(In4)
  Demux/4 -> Subsystem/32(In5)
  Demux/3 -> Subsystem/33(In6)
  Demux/2 -> Subsystem/34(In7)
  Demux/1 -> Subsystem/35(In8)
  Subsystem/1(SERIAL_OUT) -> SERIAL_OUT/1

== system gm_I2S/PISO_SHIFT_REG/MUX ==
  note: SEL=0 ==> IN1
  In1 : Inport
  In2 : Inport  Port=2
  SEL : Inport  Port=3  OutDataTypeStr=boolean
  Logical Operator : Logic  AllPortsSameDT=off  OutDataTypeStr=boolean
  Logical Operator1 : Logic  AllPortsSameDT=off  OutDataTypeStr=boolean
  Logical Operator2 : Logic  Operator=OR  AllPortsSameDT=off  OutDataTypeStr=boolean
  Logical Operator3 : Logic  Operator=NOT  AllPortsSameDT=off  OutDataTypeStr=boolean
  Out1 : Outport  VectorParamsAs1DForOutWhenUnconnected=off
  wires:
  In2/1 -> Logical Operator1/2
  Logical Operator2/1 -> Out1/1
  Logical Operator/1 -> Logical Operator2/1
  Logical Operator1/1 -> Logical Operator2/2
  Logical Operator3/1 -> Logical Operator/2
  SEL/1 -> Logical Operator1/1, Logical Operator3/1
  In1/1 -> Logical Operator/1

== system gm_I2S/PISO_SHIFT_REG/MUX1 ==
  note: SEL=0 ==> IN1
  In1 : Inport
  In2 : Inport  Port=2
  SEL : Inport  Port=3  OutDataTypeStr=boolean
  Logical Operator : Logic  AllPortsSameDT=off  OutDataTypeStr=boolean
  Logical Operator1 : Logic  AllPortsSameDT=off  OutDataTypeStr=boolean
  Logical Operator2 : Logic  Operator=OR  AllPortsSameDT=off  OutDataTypeStr=boolean
  Logical Operator3 : Logic  Operator=NOT  AllPortsSameDT=off  OutDataTypeStr=boolean
  Out1 : Outport  VectorParamsAs1DForOutWhenUnconnected=off
  wires:
  In2/1 -> Logical Operator1/2
  Logical Operator2/1 -> Out1/1
  Logical Operator/1 -> Logical Operator2/1
  Logical Operator1/1 -> Logical Operator2/2
  Logical Operator3/1 -> Logical Operator/2
  SEL/1 -> Logical Operator1/1, Logical Operator3/1
  In1/1 -> Logical Operator/1

== system gm_I2S/PISO_SHIFT_REG/MUX10 ==
  note: SEL=0 ==> IN1
  In1 : Inport
  In2 : Inport  Port=2
  SEL : Inport  Port=3  OutDataTypeStr=boolean
  Logical Operator : Logic  AllPortsSameDT=off  OutDataTypeStr=boolean
  Logical Operator1 : Logic  AllPortsSameDT=off  OutDataTypeStr=boolean
  Logical Operator2 : Logic  Operator=OR  AllPortsSameDT=off  OutDataTypeStr=boolean
  Logical Operator3 : Logic  Operator=NOT  AllPortsSameDT=off  OutDataTypeStr=boolean
  Out1 : Outport  VectorParamsAs1DForOutWhenUnconnected=off
  wires:
  In2/1 -> Logical Operator1/2
  Logical Operator2/1 -> Out1/1
  Logical Operator/1 -> Logical Operator2/1
  Logical Operator1/1 -> Logical Operator2/2
  Logical Operator3/1 -> Logical Operator/2
  SEL/1 -> Logical Operator1/1, Logical Operator3/1
  In1/1 -> Logical Operator/1

== system gm_I2S/PISO_SHIFT_REG/MUX11 ==
  note: SEL=0 ==> IN1
  In1 : Inport
  In2 : Inport  Port=2
  SEL : Inport  Port=3  OutDataTypeStr=boolean
  Logical Operator : Logic  AllPortsSameDT=off  OutDataTypeStr=boolean
  Logical Operator1 : Logic  AllPortsSameDT=off  OutDataTypeStr=boolean
  Logical Operator2 : Logic  Operator=OR  AllPortsSameDT=off  OutDataTypeStr=boolean
  Logical Operator3 : Logic  Operator=NOT  AllPortsSameDT=off  OutDataTypeStr=boolean
  Out1 : Outport  VectorParamsAs1DForOutWhenUnconnected=off
  wires:
  In2/1 -> Logical Operator1/2
  Logical Operator2/1 -> Out1/1
  Logical Operator/1 -> Logical Operator2/1
  Logical Operator1/1 -> Logical Operator2/2
  Logical Operator3/1 -> Logical Operator/2
  SEL/1 -> Logical Operator1/1, Logical Operator3/1
  In1/1 -> Logical Operator/1

== system gm_I2S/PISO_SHIFT_REG/MUX12 ==
  note: SEL=0 ==> IN1
  In1 : Inport
  In2 : Inport  Port=2
  SEL : Inport  Port=3  OutDataTypeStr=boolean
  Logical Operator : Logic  AllPortsSameDT=off  OutDataTypeStr=boolean
  Logical Operator1 : Logic  AllPortsSameDT=off  OutDataTypeStr=boolean
  Logical Operator2 : Logic  Operator=OR  AllPortsSameDT=off  OutDataTypeStr=boolean
  Logical Operator3 : Logic  Operator=NOT  AllPortsSameDT=off  OutDataTypeStr=boolean
  Out1 : Outport  VectorParamsAs1DForOutWhenUnconnected=off
  wires:
  In2/1 -> Logical Operator1/2
  Logical Operator2/1 -> Out1/1
  Logical Operator/1 -> Logical Operator2/1
  Logical Operator1/1 -> Logical Operator2/2
  Logical Operator3/1 -> Logical Operator/2
  SEL/1 -> Logical Operator1/1, Logical Operator3/1
  In1/1 -> Logical Operator/1

== system gm_I2S/PISO_SHIFT_REG/MUX13 ==
  note: SEL=0 ==> IN1
  In1 : Inport
  In2 : Inport  Port=2
  SEL : Inport  Port=3  OutDataTypeStr=boolean
  Logical Operator : Logic  AllPortsSameDT=off  OutDataTypeStr=boolean
  Logical Operator1 : Logic  AllPortsSameDT=off  OutDataTypeStr=boolean
  Logical Operator2 : Logic  Operator=OR  AllPortsSameDT=off  OutDataTypeStr=boolean
  Logical Operator3 : Logic  Operator=NOT  AllPortsSameDT=off  OutDataTypeStr=boolean
  Out1 : Outport  VectorParamsAs1DForOutWhenUnconnected=off
  wires:
  In2/1 -> Logical Operator1/2
  Logical Operator2/1 -> Out1/1
  Logical Operator/1 -> Logical Operator2/1
  Logical Operator1/1 -> Logical Operator2/2
  Logical Operator3/1 -> Logical Operator/2
  SEL/1 -> Logical Operator1/1, Logical Operator3/1
  In1/1 -> Logical Operator/1

== system gm_I2S/PISO_SHIFT_REG/MUX14 ==
  note: SEL=0 ==> IN1
  In1 : Inport
  In2 : Inport  Port=2
  SEL : Inport  Port=3  OutDataTypeStr=boolean
  Logical Operator : Logic  AllPortsSameDT=off  OutDataTypeStr=boolean
  Logical Operator1 : Logic  AllPortsSameDT=off  OutDataTypeStr=boolean
  Logical Operator2 : Logic  Operator=OR  AllPortsSameDT=off  OutDataTypeStr=boolean
  Logical Operator3 : Logic  Operator=NOT  AllPortsSameDT=off  OutDataTypeStr=boolean
  Out1 : Outport  VectorParamsAs1DForOutWhenUnconnected=off
  wires:
  In2/1 -> Logical Operator1/2
  Logical Operator2/1 -> Out1/1
  Logical Operator/1 -> Logical Operator2/1
  Logical Operator1/1 -> Logical Operator2/2
  Logical Operator3/1 -> Logical Operator/2
  SEL/1 -> Logical Operator1/1, Logical Operator3/1
  In1/1 -> Logical Operator/1

== system gm_I2S/PISO_SHIFT_REG/MUX15 ==
  note: SEL=0 ==> IN1
  In1 : Inport
  In2 : Inport  Port=2
  SEL : Inport  Port=3  OutDataTypeStr=boolean
  Logical Operator : Logic  AllPortsSameDT=off  OutDataTypeStr=boolean
  Logical Operator1 : Logic  AllPortsSameDT=off  OutDataTypeStr=boolean
  Logical Operator2 : Logic  Operator=OR  AllPortsSameDT=off  OutDataTypeStr=boolean
  Logical Operator3 : Logic  Operator=NOT  AllPortsSameDT=off  OutDataTypeStr=boolean
  Out1 : Outport  VectorParamsAs1DForOutWhenUnconnected=off
  wires:
  In2/1 -> Logical Operator1/2
  Logical Operator2/1 -> Out1/1
  Logical Operator/1 -> Logical Operator2/1
  Logical Operator1/1 -> Logical Operator2/2
  Logical Operator3/1 -> Logical Operator/2
  SEL/1 -> Logical Operator1/1, Logical Operator3/1
  In1/1 -> Logical Operator/1

== system gm_I2S/PISO_SHIFT_REG/MUX16 ==
  note: SEL=0 ==> IN1
  In1 : Inport
  In2 : Inport  Port=2
  SEL : Inport  Port=3  OutDataTypeStr=boolean
  Logical Operator : Logic  AllPortsSameDT=off  OutDataTypeStr=boolean
  Logical Operator1 : Logic  AllPortsSameDT=off  OutDataTypeStr=boolean
  Logical Operator2 : Logic  Operator=OR  AllPortsSameDT=off  OutDataTypeStr=boolean
  Logical Operator3 : Logic  Operator=NOT  AllPortsSameDT=off  OutDataTypeStr=boolean
  Out1 : Outport  VectorParamsAs1DForOutWhenUnconnected=off
  wires:
  In2/1 -> Logical Operator1/2
  Logical Operator2/1 -> Out1/1
  Logical Operator/1 -> Logical Operator2/1
  Logical Operator1/1 -> Logical Operator2/2
  Logical Operator3/1 -> Logical Operator/2
  SEL/1 -> Logical Operator1/1, Logical Operator3/1
  In1/1 -> Logical Operator/1

== system gm_I2S/PISO_SHIFT_REG/MUX17 ==
  note: SEL=0 ==> IN1
  In1 : Inport
  In2 : Inport  Port=2
  SEL : Inport  Port=3  OutDataTypeStr=boolean
  Logical Operator : Logic  AllPortsSameDT=off  OutDataTypeStr=boolean
  Logical Operator1 : Logic  AllPortsSameDT=off  OutDataTypeStr=boolean
  Logical Operator2 : Logic  Operator=OR  AllPortsSameDT=off  OutDataTypeStr=boolean
  Logical Operator3 : Logic  Operator=NOT  AllPortsSameDT=off  OutDataTypeStr=boolean
  Out1 : Outport  VectorParamsAs1DForOutWhenUnconnected=off
  wires:
  In2/1 -> Logical Operator1/2
  Logical Operator2/1 -> Out1/1
  Logical Operator/1 -> Logical Operator2/1
  Logical Operator1/1 -> Logical Operator2/2
  Logical Operator3/1 -> Logical Operator/2
  SEL/1 -> Logical Operator1/1, Logical Operator3/1
  In1/1 -> Logical Operator/1

== system gm_I2S/PISO_SHIFT_REG/MUX18 ==
  note: SEL=0 ==> IN1
  In1 : Inport
  In2 : Inport  Port=2
  SEL : Inport  Port=3  OutDataTypeStr=boolean
  Logical Operator : Logic  AllPortsSameDT=off  OutDataTypeStr=boolean
  Logical Operator1 : Logic  AllPortsSameDT=off  OutDataTypeStr=boolean
  Logical Operator2 : Logic  Operator=OR  AllPortsSameDT=off  OutDataTypeStr=boolean
  Logical Operator3 : Logic  Operator=NOT  AllPortsSameDT=off  OutDataTypeStr=boolean
  Out1 : Outport  VectorParamsAs1DForOutWhenUnconnected=off
  wires:
  In2/1 -> Logical Operator1/2
  Logical Operator2/1 -> Out1/1
  Logical Operator/1 -> Logical Operator2/1
  Logical Operator1/1 -> Logical Operator2/2
  Logical Operator3/1 -> Logical Operator/2
  SEL/1 -> Logical Operator1/1, Logical Operator3/1
  In1/1 -> Logical Operator/1

== system gm_I2S/PISO_SHIFT_REG/MUX19 ==
  note: SEL=0 ==> IN1
  In1 : Inport
  In2 : Inport  Port=2
  SEL : Inport  Port=3  OutDataTypeStr=boolean
  Logical Operator : Logic  AllPortsSameDT=off  OutDataTypeStr=boolean
  Logical Operator1 : Logic  AllPortsSameDT=off  OutDataTypeStr=boolean
  Logical Operator2 : Logic  Operator=OR  AllPortsSameDT=off  OutDataTypeStr=boolean
  Logical Operator3 : Logic  Operator=NOT  AllPortsSameDT=off  OutDataTypeStr=boolean
  Out1 : Outport  VectorParamsAs1DForOutWhenUnconnected=off
  wires:
  In2/1 -> Logical Operator1/2
  Logical Operator2/1 -> Out1/1
  Logical Operator/1 -> Logical Operator2/1
  Logical Operator1/1 -> Logical Operator2/2
  Logical Operator3/1 -> Logical Operator/2
  SEL/1 -> Logical Operator1/1, Logical Operator3/1
  In1/1 -> Logical Operator/1

== system gm_I2S/PISO_SHIFT_REG/MUX2 ==
  note: SEL=0 ==> IN1
  In1 : Inport
  In2 : Inport  Port=2
  SEL : Inport  Port=3  OutDataTypeStr=boolean
  Logical Operator : Logic  AllPortsSameDT=off  OutDataTypeStr=boolean
  Logical Operator1 : Logic  AllPortsSameDT=off  OutDataTypeStr=boolean
  Logical Operator2 : Logic  Operator=OR  AllPortsSameDT=off  OutDataTypeStr=boolean
  Logical Operator3 : Logic  Operator=NOT  AllPortsSameDT=off  OutDataTypeStr=boolean
  Out1 : Outport  VectorParamsAs1DForOutWhenUnconnected=off
  wires:
  In2/1 -> Logical Operator1/2
  Logical Operator2/1 -> Out1/1
  Logical Operator/1 -> Logical Operator2/1
  Logical Operator1/1 -> Logical Operator2/2
  Logical Operator3/1 -> Logical Operator/2
  SEL/1 -> Logical Operator1/1, Logical Operator3/1
  In1/1 -> Logical Operator/1

== system gm_I2S/PISO_SHIFT_REG/MUX20 ==
  note: SEL=0 ==> IN1
  In1 : Inport
  In2 : Inport  Port=2
  SEL : Inport  Port=3  OutDataTypeStr=boolean
  Logical Operator : Logic  AllPortsSameDT=off  OutDataTypeStr=boolean
  Logical Operator1 : Logic  AllPortsSameDT=off  OutDataTypeStr=boolean
  Logical Operator2 : Logic  Operator=OR  AllPortsSameDT=off  OutDataTypeStr=boolean
  Logical Operator3 : Logic  Operator=NOT  AllPortsSameDT=off  OutDataTypeStr=boolean
  Out1 : Outport  VectorParamsAs1DForOutWhenUnconnected=off
  wires:
  In2/1 -> Logical Operator1/2
  Logical Operator2/1 -> Out1/1
  Logical Operator/1 -> Logical Operator2/1
  Logical Operator1/1 -> Logical Operator2/2
  Logical Operator3/1 -> Logical Operator/2
  SEL/1 -> Logical Operator1/1, Logical Operator3/1
  In1/1 -> Logical Operator/1

== system gm_I2S/PISO_SHIFT_REG/MUX21 ==
  note: SEL=0 ==> IN1
  In1 : Inport
  In2 : Inport  Port=2
  SEL : Inport  Port=3  OutDataTypeStr=boolean
  Logical Operator : Logic  AllPortsSameDT=off  OutDataTypeStr=boolean
  Logical Operator1 : Logic  AllPortsSameDT=off  OutDataTypeStr=boolean
  Logical Operator2 : Logic  Operator=OR  AllPortsSameDT=off  OutDataTypeStr=boolean
  Logical Operator3 : Logic  Operator=NOT  AllPortsSameDT=off  OutDataTypeStr=boolean
  Out1 : Outport  VectorParamsAs1DForOutWhenUnconnected=off
  wires:
  In2/1 -> Logical Operator1/2
  Logical Operator2/1 -> Out1/1
  Logical Operator/1 -> Logical Operator2/1
  Logical Operator1/1 -> Logical Operator2/2
  Logical Operator3/1 -> Logical Operator/2
  SEL/1 -> Logical Operator1/1, Logical Operator3/1
  In1/1 -> Logical Operator/1

== system gm_I2S/PISO_SHIFT_REG/MUX22 ==
  note: SEL=0 ==> IN1
  In1 : Inport
  In2 : Inport  Port=2
  SEL : Inport  Port=3  OutDataTypeStr=boolean
  Logical Operator : Logic  AllPortsSameDT=off  OutDataTypeStr=boolean
  Logical Operator1 : Logic  AllPortsSameDT=off  OutDataTypeStr=boolean
  Logical Operator2 : Logic  Operator=OR  AllPortsSameDT=off  OutDataTypeStr=boolean
  Logical Operator3 : Logic  Operator=NOT  AllPortsSameDT=off  OutDataTypeStr=boolean
  Out1 : Outport  VectorParamsAs1DForOutWhenUnconnected=off
  wires:
  In2/1 -> Logical Operator1/2
  Logical Operator2/1 -> Out1/1
  Logical Operator/1 -> Logical Operator2/1
  Logical Operator1/1 -> Logical Operator2/2
  Logical Operator3/1 -> Logical Operator/2
  SEL/1 -> Logical Operator1/1, Logical Operator3/1
  In1/1 -> Logical Operator/1

== system gm_I2S/PISO_SHIFT_REG/MUX23 ==
  note: SEL=0 ==> IN1
  In1 : Inport
  In2 : Inport  Port=2
  SEL : Inport  Port=3  OutDataTypeStr=boolean
  Logical Operator : Logic  AllPortsSameDT=off  OutDataTypeStr=boolean
  Logical Operator1 : Logic  AllPortsSameDT=off  OutDataTypeStr=boolean
  Logical Operator2 : Logic  Operator=OR  AllPortsSameDT=off  OutDataTypeStr=boolean
  Logical Operator3 : Logic  Operator=NOT  AllPortsSameDT=off  OutDataTypeStr=boolean
  Out1 : Outport  VectorParamsAs1DForOutWhenUnconnected=off
  wires:
  In2/1 -> Logical Operator1/2
  Logical Operator2/1 -> Out1/1
  Logical Operator/1 -> Logical Operator2/1
  Logical Operator1/1 -> Logical Operator2/2
  Logical Operator3/1 -> Logical Operator/2
  SEL/1 -> Logical Operator1/1, Logical Operator3/1
  In1/1 -> Logical Operator/1

== system gm_I2S/PISO_SHIFT_REG/MUX24 ==
  note: SEL=0 ==> IN1
  In1 : Inport
  In2 : Inport  Port=2
  SEL : Inport  Port=3  OutDataTypeStr=boolean
  Logical Operator : Logic  AllPortsSameDT=off  OutDataTypeStr=boolean
  Logical Operator1 : Logic  AllPortsSameDT=off  OutDataTypeStr=boolean
  Logical Operator2 : Logic  Operator=OR  AllPortsSameDT=off  OutDataTypeStr=boolean
  Logical Operator3 : Logic  Operator=NOT  AllPortsSameDT=off  OutDataTypeStr=boolean
  Out1 : Outport  VectorParamsAs1DForOutWhenUnconnected=off
  wires:
  In2/1 -> Logical Operator1/2
  Logical Operator2/1 -> Out1/1
  Logical Operator/1 -> Logical Operator2/1
  Logical Operator1/1 -> Logical Operator2/2
  Logical Operator3/1 -> Logical Operator/2
  SEL/1 -> Logical Operator1/1, Logical Operator3/1
  In1/1 -> Logical Operator/1

== system gm_I2S/PISO_SHIFT_REG/MUX25 ==
  note: SEL=0 ==> IN1
  In1 : Inport
  In2 : Inport  Port=2
  SEL : Inport  Port=3  OutDataTypeStr=boolean
  Logical Operator : Logic  AllPortsSameDT=off  OutDataTypeStr=boolean
  Logical Operator1 : Logic  AllPortsSameDT=off  OutDataTypeStr=boolean
  Logical Operator2 : Logic  Operator=OR  AllPortsSameDT=off  OutDataTypeStr=boolean
  Logical Operator3 : Logic  Operator=NOT  AllPortsSameDT=off  OutDataTypeStr=boolean
  Out1 : Outport  VectorParamsAs1DForOutWhenUnconnected=off
  wires:
  In2/1 -> Logical Operator1/2
  Logical Operator2/1 -> Out1/1
  Logical Operator/1 -> Logical Operator2/1
  Logical Operator1/1 -> Logical Operator2/2
  Logical Operator3/1 -> Logical Operator/2
  SEL/1 -> Logical Operator1/1, Logical Operator3/1
  In1/1 -> Logical Operator/1

== system gm_I2S/PISO_SHIFT_REG/MUX26 ==
  note: SEL=0 ==> IN1
  In1 : Inport
  In2 : Inport  Port=2
  SEL : Inport  Port=3  OutDataTypeStr=boolean
  Logical Operator : Logic  AllPortsSameDT=off  OutDataTypeStr=boolean
  Logical Operator1 : Logic  AllPortsSameDT=off  OutDataTypeStr=boolean
  Logical Operator2 : Logic  Operator=OR  AllPortsSameDT=off  OutDataTypeStr=boolean
  Logical Operator3 : Logic  Operator=NOT  AllPortsSameDT=off  OutDataTypeStr=boolean
  Out1 : Outport  VectorParamsAs1DForOutWhenUnconnected=off
  wires:
  In2/1 -> Logical Operator1/2
  Logical Operator2/1 -> Out1/1
  Logical Operator/1 -> Logical Operator2/1
  Logical Operator1/1 -> Logical Operator2/2
  Logical Operator3/1 -> Logical Operator/2
  SEL/1 -> Logical Operator1/1, Logical Operator3/1
  In1/1 -> Logical Operator/1

== system gm_I2S/PISO_SHIFT_REG/MUX27 ==
  note: SEL=0 ==> IN1
  In1 : Inport
  In2 : Inport  Port=2
  SEL : Inport  Port=3  OutDataTypeStr=boolean
  Logical Operator : Logic  AllPortsSameDT=off  OutDataTypeStr=boolean
  Logical Operator1 : Logic  AllPortsSameDT=off  OutDataTypeStr=boolean
  Logical Operator2 : Logic  Operator=OR  AllPortsSameDT=off  OutDataTypeStr=boolean
  Logical Operator3 : Logic  Operator=NOT  AllPortsSameDT=off  OutDataTypeStr=boolean
  Out1 : Outport  VectorParamsAs1DForOutWhenUnconnected=off
  wires:
  In2/1 -> Logical Operator1/2
  Logical Operator2/1 -> Out1/1
  Logical Operator/1 -> Logical Operator2/1
  Logical Operator1/1 -> Logical Operator2/2
  Logical Operator3/1 -> Logical Operator/2
  SEL/1 -> Logical Operator1/1, Logical Operator3/1
  In1/1 -> Logical Operator/1

== system gm_I2S/PISO_SHIFT_REG/MUX28 ==
  note: SEL=0 ==> IN1
  In1 : Inport
  In2 : Inport  Port=2
  SEL : Inport  Port=3  OutDataTypeStr=boolean
  Logical Operator : Logic  AllPortsSameDT=off  OutDataTypeStr=boolean
  Logical Operator1 : Logic  AllPortsSameDT=off  OutDataTypeStr=boolean
  Logical Operator2 : Logic  Operator=OR  AllPortsSameDT=off  OutDataTypeStr=boolean
  Logical Operator3 : Logic  Operator=NOT  AllPortsSameDT=off  OutDataTypeStr=boolean
  Out1 : Outport  VectorParamsAs1DForOutWhenUnconnected=off
  wires:
  In2/1 -> Logical Operator1/2
  Logical Operator2/1 -> Out1/1
  Logical Operator/1 -> Logical Operator2/1
  Logical Operator1/1 -> Logical Operator2/2
  Logical Operator3/1 -> Logical Operator/2
  SEL/1 -> Logical Operator1/1, Logical Operator3/1
  In1/1 -> Logical Operator/1

== system gm_I2S/PISO_SHIFT_REG/MUX29 ==
  note: SEL=0 ==> IN1
  In1 : Inport
  In2 : Inport  Port=2
  SEL : Inport  Port=3  OutDataTypeStr=boolean
  Logical Operator : Logic  AllPortsSameDT=off  OutDataTypeStr=boolean
  Logical Operator1 : Logic  AllPortsSameDT=off  OutDataTypeStr=boolean
  Logical Operator2 : Logic  Operator=OR  AllPortsSameDT=off  OutDataTypeStr=boolean
  Logical Operator3 : Logic  Operator=NOT  AllPortsSameDT=off  OutDataTypeStr=boolean
  Out1 : Outport  VectorParamsAs1DForOutWhenUnconnected=off
  wires:
  In2/1 -> Logical Operator1/2
  Logical Operator2/1 -> Out1/1
  Logical Operator/1 -> Logical Operator2/1
  Logical Operator1/1 -> Logical Operator2/2
  Logical Operator3/1 -> Logical Operator/2
  SEL/1 -> Logical Operator1/1, Logical Operator3/1
  In1/1 -> Logical Operator/1

== system gm_I2S/PISO_SHIFT_REG/MUX3 ==
  note: SEL=0 ==> IN1
  In1 : Inport
  In2 : Inport  Port=2
  SEL : Inport  Port=3  OutDataTypeStr=boolean
  Logical Operator : Logic  AllPortsSameDT=off  OutDataTypeStr=boolean
  Logical Operator1 : Logic  AllPortsSameDT=off  OutDataTypeStr=boolean
  Logical Operator2 : Logic  Operator=OR  AllPortsSameDT=off  OutDataTypeStr=boolean
  Logical Operator3 : Logic  Operator=NOT  AllPortsSameDT=off  OutDataTypeStr=boolean
  Out1 : Outport  VectorParamsAs1DForOutWhenUnconnected=off
  wires:
  In2/1 -> Logical Operator1/2
  Logical Operator2/1 -> Out1/1
  Logical Operator/1 -> Logical Operator2/1
  Logical Operator1/1 -> Logical Operator2/2
  Logical Operator3/1 -> Logical Operator/2
  SEL/1 -> Logical Operator1/1, Logical Operator3/1
  In1/1 -> Logical Operator/1

== system gm_I2S/PISO_SHIFT_REG/MUX30 ==
  note: SEL=0 ==> IN1
  In1 : Inport
  In2 : Inport  Port=2
  SEL : Inport  Port=3  OutDataTypeStr=boolean
  Logical Operator : Logic  AllPortsSameDT=off  OutDataTypeStr=boolean
  Logical Operator1 : Logic  AllPortsSameDT=off  OutDataTypeStr=boolean
  Logical Operator2 : Logic  Operator=OR  AllPortsSameDT=off  OutDataTypeStr=boolean
  Logical Operator3 : Logic  Operator=NOT  AllPortsSameDT=off  OutDataTypeStr=boolean
  Out1 : Outport  VectorParamsAs1DForOutWhenUnconnected=off
  wires:
  In2/1 -> Logical Operator1/2
  Logical Operator2/1 -> Out1/1
  Logical Operator/1 -> Logical Operator2/1
  Logical Operator1/1 -> Logical Operator2/2
  Logical Operator3/1 -> Logical Operator/2
  SEL/1 -> Logical Operator1/1, Logical Operator3/1
  In1/1 -> Logical Operator/1

== system gm_I2S/PISO_SHIFT_REG/MUX31 ==
  note: SEL=0 ==> IN1
  In1 : Inport
  In2 : Inport  Port=2
  SEL : Inport  Port=3  OutDataTypeStr=boolean
  Logical Operator : Logic  AllPortsSameDT=off  OutDataTypeStr=boolean
  Logical Operator1 : Logic  AllPortsSameDT=off  OutDataTypeStr=boolean
  Logical Operator2 : Logic  Operator=OR  AllPortsSameDT=off  OutDataTypeStr=boolean
  Logical Operator3 : Logic  Operator=NOT  AllPortsSameDT=off  OutDataTypeStr=boolean
  Out1 : Outport  VectorParamsAs1DForOutWhenUnconnected=off
  wires:
  In2/1 -> Logical Operator1/2
  Logical Operator2/1 -> Out1/1
  Logical Operator/1 -> Logical Operator2/1
  Logical Operator1/1 -> Logical Operator2/2
  Logical Operator3/1 -> Logical Operator/2
  SEL/1 -> Logical Operator1/1, Logical Operator3/1
  In1/1 -> Logical Operator/1

== system gm_I2S/PISO_SHIFT_REG/MUX4 ==
  note: SEL=0 ==> IN1
  In1 : Inport
  In2 : Inport  Port=2
  SEL : Inport  Port=3  OutDataTypeStr=boolean
  Logical Operator : Logic  AllPortsSameDT=off  OutDataTypeStr=boolean
  Logical Operator1 : Logic  AllPortsSameDT=off  OutDataTypeStr=boolean
  Logical Operator2 : Logic  Operator=OR  AllPortsSameDT=off  OutDataTypeStr=boolean
  Logical Operator3 : Logic  Operator=NOT  AllPortsSameDT=off  OutDataTypeStr=boolean
  Out1 : Outport  VectorParamsAs1DForOutWhenUnconnected=off
  wires:
  In2/1 -> Logical Operator1/2
  Logical Operator2/1 -> Out1/1
  Logical Operator/1 -> Logical Operator2/1
  Logical Operator1/1 -> Logical Operator2/2
  Logical Operator3/1 -> Logical Operator/2
  SEL/1 -> Logical Operator1/1, Logical Operator3/1
  In1/1 -> Logical Operator/1

== system gm_I2S/PISO_SHIFT_REG/MUX5 ==
  note: SEL=0 ==> IN1
  In1 : Inport
  In2 : Inport  Port=2
  SEL : Inport  Port=3  OutDataTypeStr=boolean
  Logical Operator : Logic  AllPortsSameDT=off  OutDataTypeStr=boolean
  Logical Operator1 : Logic  AllPortsSameDT=off  OutDataTypeStr=boolean
  Logical Operator2 : Logic  Operator=OR  AllPortsSameDT=off  OutDataTypeStr=boolean
  Logical Operator3 : Logic  Operator=NOT  AllPortsSameDT=off  OutDataTypeStr=boolean
  Out1 : Outport  VectorParamsAs1DForOutWhenUnconnected=off
  wires:
  In2/1 -> Logical Operator1/2
  Logical Operator2/1 -> Out1/1
  Logical Operator/1 -> Logical Operator2/1
  Logical Operator1/1 -> Logical Operator2/2
  Logical Operator3/1 -> Logical Operator/2
  SEL/1 -> Logical Operator1/1, Logical Operator3/1
  In1/1 -> Logical Operator/1

== system gm_I2S/PISO_SHIFT_REG/MUX6 ==
  note: SEL=0 ==> IN1
  In1 : Inport
  In2 : Inport  Port=2
  SEL : Inport  Port=3  OutDataTypeStr=boolean
  Logical Operator : Logic  AllPortsSameDT=off  OutDataTypeStr=boolean
  Logical Operator1 : Logic  AllPortsSameDT=off  OutDataTypeStr=boolean
  Logical Operator2 : Logic  Operator=OR  AllPortsSameDT=off  OutDataTypeStr=boolean
  Logical Operator3 : Logic  Operator=NOT  AllPortsSameDT=off  OutDataTypeStr=boolean
  Out1 : Outport  VectorParamsAs1DForOutWhenUnconnected=off
  wires:
  In2/1 -> Logical Operator1/2
  Logical Operator2/1 -> Out1/1
  Logical Operator/1 -> Logical Operator2/1
  Logical Operator1/1 -> Logical Operator2/2
  Logical Operator3/1 -> Logical Operator/2
  SEL/1 -> Logical Operator1/1, Logical Operator3/1
  In1/1 -> Logical Operator/1

== system gm_I2S/PISO_SHIFT_REG/MUX7 ==
  note: SEL=0 ==> IN1
  In1 : Inport
  In2 : Inport  Port=2
  SEL : Inport  Port=3  OutDataTypeStr=boolean
  Logical Operator : Logic  AllPortsSameDT=off  OutDataTypeStr=boolean
  Logical Operator1 : Logic  AllPortsSameDT=off  OutDataTypeStr=boolean
  Logical Operator2 : Logic  Operator=OR  AllPortsSameDT=off  OutDataTypeStr=boolean
  Logical Operator3 : Logic  Operator=NOT  AllPortsSameDT=off  OutDataTypeStr=boolean
  Out1 : Outport  VectorParamsAs1DForOutWhenUnconnected=off
  wires:
  In2/1 -> Logical Operator1/2
  Logical Operator2/1 -> Out1/1
  Logical Operator/1 -> Logical Operator2/1
  Logical Operator1/1 -> Logical Operator2/2
  Logical Operator3/1 -> Logical Operator/2
  SEL/1 -> Logical Operator1/1, Logical Operator3/1
  In1/1 -> Logical Operator/1

== system gm_I2S/PISO_SHIFT_REG/MUX8 ==
  note: SEL=0 ==> IN1
  In1 : Inport
  In2 : Inport  Port=2
  SEL : Inport  Port=3  OutDataTypeStr=boolean
  Logical Operator : Logic  AllPortsSameDT=off  OutDataTypeStr=boolean
  Logical Operator1 : Logic  AllPortsSameDT=off  OutDataTypeStr=boolean
  Logical Operator2 : Logic  Operator=OR  AllPortsSameDT=off  OutDataTypeStr=boolean
  Logical Operator3 : Logic  Operator=NOT  AllPortsSameDT=off  OutDataTypeStr=boolean
  Out1 : Outport  VectorParamsAs1DForOutWhenUnconnected=off
  wires:
  In2/1 -> Logical Operator1/2
  Logical Operator2/1 -> Out1/1
  Logical Operator/1 -> Logical Operator2/1
  Logical Operator1/1 -> Logical Operator2/2
  Logical Operator3/1 -> Logical Operator/2
  SEL/1 -> Logical Operator1/1, Logical Operator3/1
  In1/1 -> Logical Operator/1
